simulink model "BE2et5_simu_int"  (R2018b)
settings: Solver=VariableStepAuto  StartTime=0.0  StopTime=120  RelTol=1e-3
values from neighbouring files (symbols this model uses):
  A = [1.5 0 0 0; 0 3 0 0; 0 0 0.5 0; 0 0 0 0.9]    [BE1.m]    (also in BE2a5.m = [a 0 ; (3*alpha0*v0^2)/(J*w0) (-alpha0*v0^3)/(J*w0^2)])
  B = [1 2; 1 2; 0 0; 1 2]    [BE1.m]    (also in BE2a5.m = [0 ; -Ke/J])
  C = [1 1 1 0; 0 1 3 1]    [BE1.m]    (also in BE2a5.m = [0  1])
  F = inv(R + B'*P*B)*B'*P*A    [BE1.m]    (also in BE2a5.m = lqr(sysC, Q, R))
  Fe = Fi(1,1:2)    [BE2a5.m]
  H = Fi(1,3)    [BE2a5.m]
  K = lqr(A',C',W,V)'    [BE2a5.m]
  L = [-lambda/r 1]    [BE2a5.m]
  x0 = [2 2 2 2]'    [BE1.m]    (also in BE2a5.m = [v0, w0])
settings Model: Creator=piffercg  LastModifiedBy=piffercg

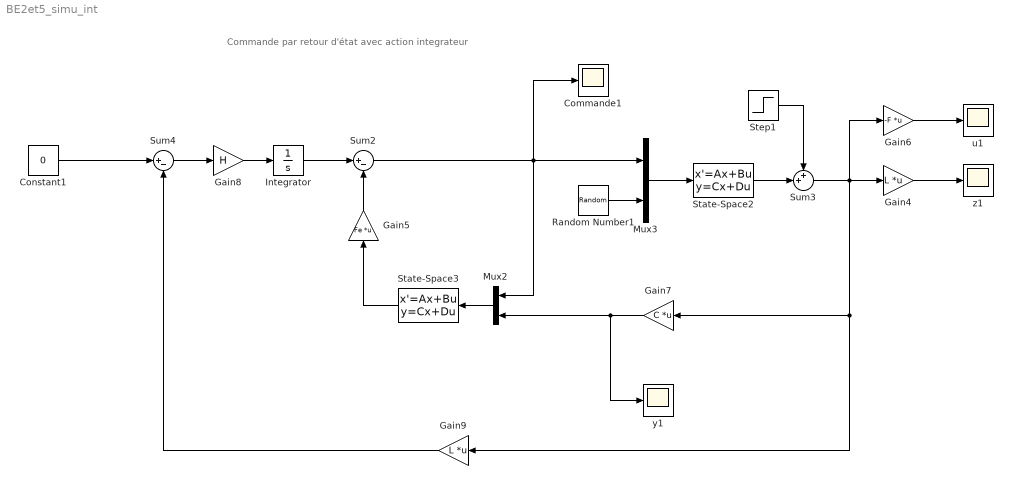
== system BE2et5_simu_int ==
  note: Commande par retour d'état avec action integrateur
  Commande1 : Scope
  Constant1 : Constant  Value=0
  Gain4 : Gain  Gain=L  Multiplication=Matrix(K*u) (u vector)
  Gain5 : Gain  Gain=Fe  Multiplication=Matrix(K*u)
  Gain6 : Gain  Gain=-F  Multiplication=Matrix(K*u) (u vector)
  Gain7 : Gain  Gain=C  Multiplication=Matrix(K*u) (u vector)
  Gain8 : Gain  Gain=H
  Gain9 : Gain  Gain=L  Multiplication=Matrix(K*u)
  Integrator : Integrator
  Mux2 : Mux  Inputs=2
  Mux3 : Mux  Inputs=2
  Random Number1 : RandomNumber  SampleTime=1
  State-Space2 : StateSpace  A=A  B=[B E]  C=eye(2)  D=[0 0; 0 0]  InitialCondition=x0
  State-Space3 : StateSpace  A=A-K*C  B=[B E]  C=eye(2)  D=[0 0; 0 0]  InitialCondition=0
  Step1 : Step  Time=50  After=5  SampleTime=0
  Sum2 : Sum  Inputs=|+-
  Sum3 : Sum  Inputs=++|
  Sum4 : Sum  Inputs=|+-
  u1 : Scope
  y1 : Scope
  z1 : Scope
  wires:
  Gain7/1 -> y1/1, Mux2/2
  Gain9/1 -> Sum4/2
  Sum2/1 -> Mux2/1, Commande1/1, Mux3/1
  Constant1/1 -> Sum4/1
  State-Space3/1 -> Gain5/1
  Random Number1/1 -> Mux3/2
  Sum4/1 -> Gain8/1
  Integrator/1 -> Sum2/1
  State-Space2/1 -> Sum3/2
  Step1/1 -> Sum3/1
  Sum3/1 -> Gain9/1, Gain7/1, Gain6/1, Gain4/1
  Gain4/1 -> z1/1
  Gain6/1 -> u1/1
  Gain5/1 -> Sum2/2
  Mux2/1 -> State-Space3/1
  Gain8/1 -> Integrator/1
  Mux3/1 -> State-Space2/1
